simulink model "sim_chua_fl"  (R2017b)
settings: Solver=ode4  StartTime=0.0  StopTime=tfin  FixedStep=0.1  RelTol=1e-3
values from neighbouring files (symbols this model uses):
  C = [1 0 0]    [main_chua_fl.m]
  x0 = randn(3,1)*0    [main_chua_fl.m]
undefined symbols (not defined in the file or in its folder): fg_chua, u_chua
libraries: cstblocks x1
settings Model: Creator=carlonovara  LastModifiedBy=carlonovara
settings CodeAppCC: StateflowObjectComments=on

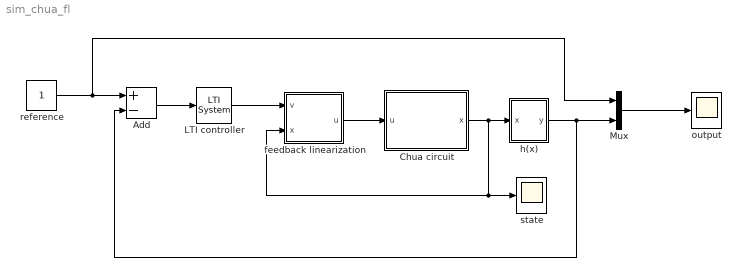
== system sim_chua_fl ==
  Add : Sum  Inputs=+-
  Chua circuit : Subsystem
  LTI controller : cstblocks/LTI System  sys=K  IC=[]
  Mux : Mux  Inputs=2
  feedback linearization : Subsystem
  h(x) : Subsystem
  output : Scope
  reference : Constant
  state : Scope
  wires:
  Chua circuit/1(x) -> h(x)/1(x), state/1, feedback linearization/2(x)
  feedback linearization/1(u) -> Chua circuit/1(u)
  h(x)/1(y) -> Add/2, Mux/2
  Add/1 -> LTI controller/1
  LTI controller/1 -> feedback linearization/1(v)
  Mux/1 -> output/1
  reference/1 -> Mux/1, Add/1

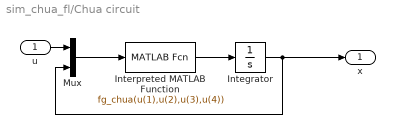
== system sim_chua_fl/Chua circuit ==
  u : Inport
  Integrator : Integrator  InitialCondition=x0
  Interpreted MATLAB Function : MATLABFcn  MATLABFcn=fg_chua(u(1),u(2),u(3),u(4))  OutputDimensions=3
  Mux : Mux  Inputs=2
  x : Outport
  wires:
  u/1 -> Mux/1
  Interpreted MATLAB Function/1 -> Integrator/1
  Integrator/1 -> Mux/2, x/1
  Mux/1 -> Interpreted MATLAB Function/1

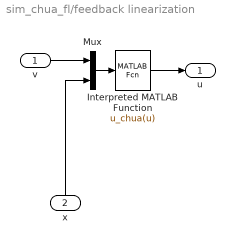
== system sim_chua_fl/feedback linearization ==
  v : Inport
  x : Inport  Port=2
  Interpreted MATLAB Function : MATLABFcn  MATLABFcn=u_chua(u)
  Mux : Mux  Inputs=2
  u : Outport
  wires:
  x/1 -> Mux/2
  Mux/1 -> Interpreted MATLAB Function/1
  Interpreted MATLAB Function/1 -> u/1
  v/1 -> Mux/1

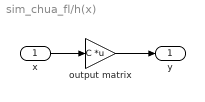
== system sim_chua_fl/h(x) ==
  x : Inport
  output matrix : Gain  Gain=C  Multiplication=Matrix(K*u)
  y : Outport
  wires:
  x/1 -> output matrix/1
  output matrix/1 -> y/1
